simulink model "BD_SER_saber_cosim"  (Simulink 4.1.1)
settings: Solver=ode1  SolverMode=SingleTasking  StartTime=0.0  StopTime=max(cyc_mph(:,1))  FixedStep=1  MaxStep=1  RelTol=1e-3  AbsTol=1e-3
undefined symbols (not defined in the file): cs_fc_off2regen_pwr, cs_fc_spd_setpt_fun, cs_fc_trq_setpt_fun, cs_hi_soc, cs_lo_soc, cyc_mph, ess_max_volts_fun, ess_min_volts_fun, ess_on, ex_calc, fc_emis, fc_map_spd, fc_max_trq, fc_on, fc_spd_scale, fc_trq_scale, fd_ratio, gb_dnshift_load, gb_dnshift_spd, gb_gears_num, gb_num_init, gb_ratio, gb_shift_delay, gb_upshift_load, gb_upshift_spd, gc_map_spd, gc_max_trq, gc_spd_scale, gc_trq_scale, mc_map_spd, mc_max_trq, mc_spd_scale, mc_trq_scale, tc_gc_to_fc_ratio_fun, time_step, tx_speed_dep, vc_idle_bool, vc_idle_spd, wh_radius
libraries: lib_cosimulation x10, lib_outputs x8, lib_controls x5, lib_wheel x2, lib_help x2, lib_transmission x2, lib_accessory x2, lib_interactive x1, lib_drive_cycle x1, lib_exhaust x1, lib_fuel_converter x1, lib_vehicle x1
(part 2 of 2)

== system BD_SER_saber_cosim/Cosimulate Elect/Motor RPM Req/Enabled Subsystem ==
  In1 : Inport  Port=1  LatchInput=off
  Enable : EnablePort
  Out1 : Outport  Port=1
  wires:
  In1/1 -> Out1/1

== system BD_SER_saber_cosim/Cosimulate Elect/Motor Trq Req/Enabled Subsystem ==
  In1 : Inport  Port=1  LatchInput=off
  Enable : EnablePort
  Out1 : Outport  Port=1  InitialOutput=0
  wires:
  In1/1 -> Out1/1

== system BD_SER_saber_cosim/Cosimulate Elect/Series cosim output gotos/Saber_ess2_outputs ==
  In1 : Inport  Port=1  LatchInput=off
  Saber_pb2 : lib_outputs/Saber_pb2
      settings: RTWFcnNameOpts=Auto  RTWFileNameOpts=Auto
  wires:
  In1/1 -> Saber_pb2/1

== system BD_SER_saber_cosim/Cosimulate Elect/Series cosim output gotos/Saber_ess_outputs ==
  In1 : Inport  Port=1  LatchInput=off
  Saber_rint : lib_outputs/Saber_rint
      settings: RTWFcnNameOpts=Auto  RTWFileNameOpts=Auto
  wires:
  In1/1 -> Saber_rint/1

== system BD_SER_saber_cosim/series hybrid control stategy  <cs>/FC on mod/Charge to hi soc: 1 Discharge to lo soc: 0 ==
  In1 : Inport  Port=1  LatchInput=off
  Trigger : TriggerPort  TriggerType=rising  OutputDataType=auto
  Out1 : Outport  Port=1
  wires:
  In1/1 -> Out1/1

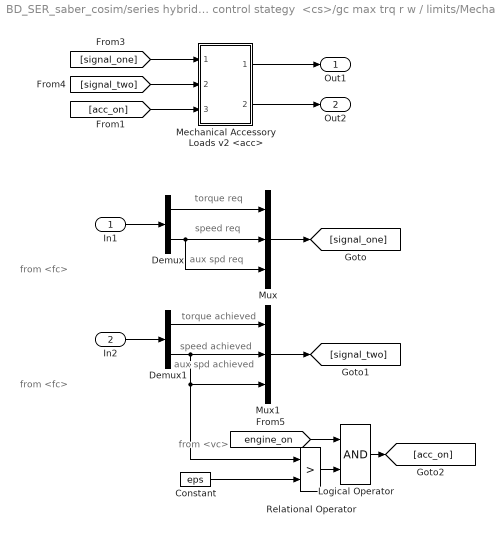
== system BD_SER_saber_cosim/series hybrid control stategy  <cs>/gc max trq r w / limits/Mechanical Accessory Loads <acc> ==
  note: from <fc>
  note: from <fc>
  note: torque req
  note: speed req
  note: aux spd req
  note: torque achieved
  note: speed achieved
  note: aux spd achieved
  note: from <vc>
  In1 : Inport  Port=1  LatchInput=off
  In2 : Inport  Port=2  LatchInput=off
  Constant : Constant  Value=eps
  Demux : Demux  Outputs=2  BusSelectionMode=off
  Demux1 : Demux  Outputs=2  BusSelectionMode=off
  Logical Operator : Logic  Operator=AND  Inputs=2
  Mechanical Accessory Loads v2 <acc> : Subsystem  AncestorBlock=lib_accessory/Mechanical Accessory Loads v2 <acc>  mask{load_on=not(ess_on)*1, acc_max_spd=inf, acc_min_spd=(vc_idle_spd*vc_idle_bool)+eps, ic_mech_trq=0, ic_mech_pwr=0}
      mask prompts: load_on "Electrical Load Status: 1 on; 0 off"; acc_max_spd "maximum shaft speed for aux. (rad/s)"; acc_min_spd "minimum shaft speed for aux. (rad/s)"; ic_mech_trq "Initial Mechanical Torque of the Accessory Loads (Nm)"; ic_mech_pwr "Initial Mechanical Auxiliary Load Power (W)"
      settings: RTWFcnNameOpts=Auto  RTWFileNameOpts=Auto
      mask Display: image(imread('bdi_acc_pic.bmp'))
  Mux : Mux  Inputs=3
  Mux1 : Mux  Inputs=3
  Relational Operator : RelationalOperator  Operator=>
  Out1 : Outport  Port=1
  Out2 : Outport  Port=2
  wires:
  [signal_one] -> Mechanical Accessory Loads v2 <acc>/1("requested shaft T and w, out to the driveline  (Nm ; rad/s; rad/s)")
  Mechanical Accessory Loads v2 <acc>/1("requested shaft and belt T and w, in from the prime mover (Nm ; rad/s)") -> Out1/1
  Mechanical Accessory Loads v2 <acc>/2("achieved shaft T and w, out to the driveline (Nm ; rad/s)") -> Out2/1
  [signal_two] -> Mechanical Accessory Loads v2 <acc>/2("achieved shaft and belt T and w, in from the prime mover (Nm ; rad/s)")
  [acc_on] -> Mechanical Accessory Loads v2 <acc>/3(accessory on/off)
  Mux/1 -> [signal_one]
  In1/1 -> Demux/1
  Demux/1 -> Mux/1
  Demux/2 -> Mux/2, Mux/3
  Mux1/1 -> [signal_two]
  In2/1 -> Demux1/1
  Demux1/1 -> Mux1/1
  Demux1/2 -> Mux1/2, Mux1/3, Relational Operator/1
  Constant/1 -> Relational Operator/2
  [engine_on] -> Logical Operator/1
  Relational Operator/1 -> Logical Operator/2
  Logical Operator/1 -> [acc_on]

== system BD_SER_saber_cosim/<vc> series/gearbox control for series  HV and EV/downshift  command/load fraction ==
  In1 : Inport  Port=1  LatchInput=off
  S-Function : S-Function  FunctionName=sfun_gearbox  Parameters=load, spd  PortCounts=[]  SFunctionModules=''
  Out1 : Outport  Port=1  InitialOutput=0
  wires:
  S-Function/1 -> Out1/1
  In1/1 -> S-Function/1

== system BD_SER_saber_cosim/<vc> series/gearbox control for series  HV and EV/gearbox speed estimator/Block NOTES ==
  note: The requested motor speed is replaced by an estimate of the
      | engine's previous speed whenever the vehicle missed the trace
      |  by more than 1 mph on the last time step.

== system BD_SER_saber_cosim/<vc> series/gearbox control for series  HV and EV/gearbox speed estimator/dt ==
  Clock : Clock
      settings: DisplayTime=off  Decimation=10
  Memory1 : Memory  X0=-1  InheritSampleTime=off
      settings: RTWStateStorageClass=Auto
  Sum4 : Sum  Inputs=+-  SaturateOnIntegerOverflow=on
  Out1 : Outport  Port=1  InitialOutput=0
  wires:
  Clock/1 -> Sum4/1, Memory1/1
  Memory1/1 -> Sum4/2
  Sum4/1 -> Out1/1

== system BD_SER_saber_cosim/<vc> series/gearbox control for series  HV and EV/shifting1/time since last shift ==
  in_1 : Inport  Port=1  LatchInput=off
  just shifted : Subsystem
      settings: RTWFcnNameOpts=Auto  RTWFileNameOpts=Auto
      mask Display: disp('just\nshifted')
  timer : Subsystem
      settings: RTWFcnNameOpts=Auto  RTWFileNameOpts=Auto
      mask Display: disp('timer')
  out_1 : Outport  Port=1  InitialOutput=0
  wires:
  timer/1(time) -> out_1/1
  just shifted/1(out_1) -> timer/1(trigger)
  in_1/1 -> just shifted/1(in_1)

== system BD_SER_saber_cosim/<vc> series/gearbox control for series  HV and EV/upshift  command/load fraction ==
  In1 : Inport  Port=1  LatchInput=off
  S-Function : S-Function  FunctionName=sfun_gearbox  Parameters=load, spd  PortCounts=[]  SFunctionModules=''
  Out1 : Outport  Port=1  InitialOutput=0
  wires:
  S-Function/1 -> Out1/1
  In1/1 -> S-Function/1

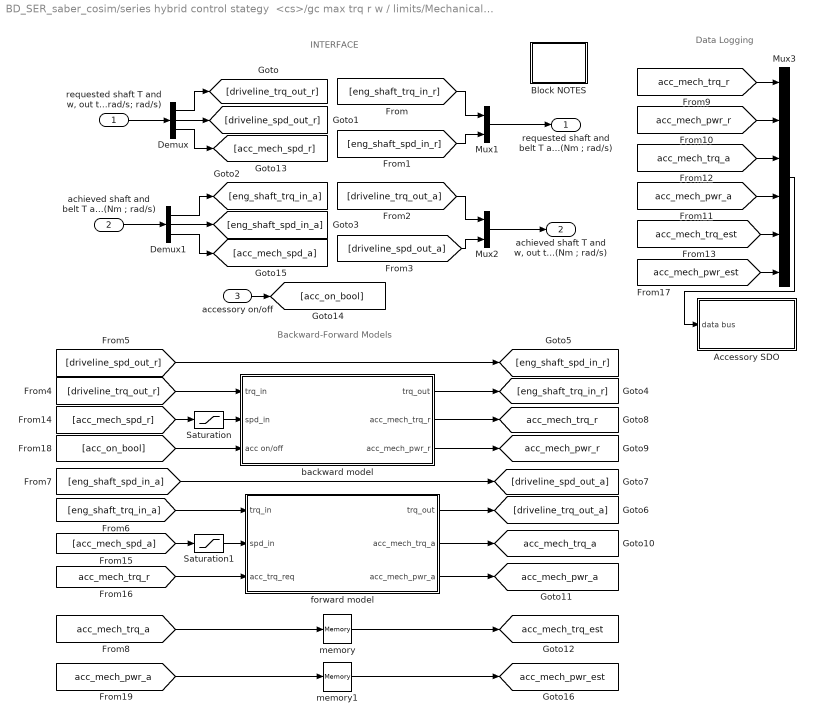
== system BD_SER_saber_cosim/series hybrid control stategy  <cs>/gc max trq r w / limits/Mechanical Accessory Loads <acc>/Mechanical Accessory Loads v2 <acc> ==
  note: Data Logging
  note: Backward-Forward Models
  note: INTERFACE
  "requested shaft T and w, out to the driveline  (Nm ; rad/s; rad/s)" : Inport  Port=1  LatchInput=off
  "achieved shaft and belt T and w, in from the prime mover (Nm ; rad/s)" : Inport  Port=2  LatchInput=off
  accessory on/off : Inport  Port=3  LatchInput=off
  Accessory SDO : Subsystem
      settings: RTWFcnNameOpts=Auto  RTWFileNameOpts=Auto
  Block NOTES : Subsystem
      settings: RTWFcnNameOpts=Auto  RTWFileNameOpts=Auto
      mask Display: disp('Block\nNOTES')
  Demux : Demux  Outputs=3  BusSelectionMode=off
  Demux1 : Demux  Outputs=3  BusSelectionMode=off
  Mux1 : Mux  Inputs=2
  Mux2 : Mux  Inputs=2
  Mux3 : Mux  Inputs=6
  Saturation : Saturate  UpperLimit=acc_max_spd  LowerLimit=acc_min_spd  LinearizeAsGain=on
  Saturation1 : Saturate  UpperLimit=acc_max_spd  LowerLimit=acc_min_spd  LinearizeAsGain=on
  backward model : Subsystem
      settings: RTWFcnNameOpts=Auto  RTWFileNameOpts=Auto
  forward model : Subsystem
      settings: RTWFcnNameOpts=Auto  RTWFileNameOpts=Auto
  memory : Memory  X0=ic_mech_trq  InheritSampleTime=off
      settings: RTWStateStorageClass=Auto
  memory1 : Memory  X0=ic_mech_pwr  InheritSampleTime=off
      settings: RTWStateStorageClass=Auto
  "requested shaft and belt T and w, in from the prime mover (Nm ; rad/s)" : Outport  Port=1
  "achieved shaft T and w, out to the driveline (Nm ; rad/s)" : Outport  Port=2
  tag scope: acc_mech_pwr_a=global, acc_mech_pwr_est=global, acc_mech_pwr_r=global, acc_mech_trq_a=global, acc_mech_trq_est=global, acc_mech_trq_r=global
  wires:
  [acc_mech_pwr_a] -> memory1/1
  [acc_mech_trq_a] -> memory/1
  memory1/1 -> [acc_mech_pwr_est]
  memory/1 -> [acc_mech_trq_est]
  [acc_mech_pwr_est] -> Mux3/6
  Demux/3 -> [acc_mech_spd_r]
  Demux1/3 -> [acc_mech_spd_a]
  [acc_mech_trq_r] -> forward model/3(acc_trq_req)
  Saturation/1 -> backward model/2(spd_in)
  [acc_mech_spd_r] -> Saturation/1
  Saturation1/1 -> forward model/2(spd_in)
  [acc_mech_spd_a] -> Saturation1/1
  forward model/3(acc_mech_pwr_a) -> [acc_mech_pwr_a]
  forward model/2(acc_mech_trq_a) -> [acc_mech_trq_a]
  forward model/1(trq_out) -> [driveline_trq_out_a]
  [acc_on_bool] -> backward model/3(acc on/off)
  accessory on/off/1 -> [acc_on_bool]
  [eng_shaft_trq_in_a] -> forward model/1(trq_in)
  [acc_mech_pwr_a] -> Mux3/4
  [acc_mech_trq_a] -> Mux3/3
  [eng_shaft_spd_in_a] -> [driveline_spd_out_a]
  [driveline_spd_out_r] -> [eng_shaft_spd_in_r]
  [acc_mech_trq_est] -> Mux3/5
  Mux3/1 -> Accessory SDO/1(data bus)
  [acc_mech_pwr_r] -> Mux3/2
  [acc_mech_trq_r] -> Mux3/1
  backward model/1(trq_out) -> [eng_shaft_trq_in_r]
  [driveline_trq_out_r] -> backward model/1(trq_in)
  backward model/3(acc_mech_pwr_r) -> [acc_mech_pwr_r]
  backward model/2(acc_mech_trq_r) -> [acc_mech_trq_r]
  [driveline_spd_out_a] -> Mux2/2
  [driveline_trq_out_a] -> Mux2/1
  Mux2/1 -> "achieved shaft T and w, out to the driveline (Nm ; rad/s)"/1
  [eng_shaft_spd_in_r] -> Mux1/2
  [eng_shaft_trq_in_r] -> Mux1/1
  Mux1/1 -> "requested shaft and belt T and w, in from the prime mover (Nm ; rad/s)"/1
  Demux1/2 -> [eng_shaft_spd_in_a]
  Demux1/1 -> [eng_shaft_trq_in_a]
  "achieved shaft and belt T and w, in from the prime mover (Nm ; rad/s)"/1 -> Demux1/1
  Demux/2 -> [driveline_spd_out_r]
  Demux/1 -> [driveline_trq_out_r]
  "requested shaft T and w, out to the driveline  (Nm ; rad/s; rad/s)"/1 -> Demux/1

== system BD_SER_saber_cosim/<vc> series/gearbox control for series  HV and EV/shifting1/time since last shift/just shifted ==
  in_1 : Inport  Port=1  LatchInput=off
  Memory : Memory  X0=1  InheritSampleTime=off
      settings: RTWStateStorageClass=Auto
  Relational Operator : RelationalOperator  Operator=~=
  out_1 : Outport  Port=1  InitialOutput=0
  wires:
  in_1/1 -> Memory/1, Relational Operator/2
  Memory/1 -> Relational Operator/1
  Relational Operator/1 -> out_1/1

== system BD_SER_saber_cosim/<vc> series/gearbox control for series  HV and EV/shifting1/time since last shift/timer ==
  trigger : Inport  Port=1  LatchInput=off
  Constant : Constant  Value=1
  Constant1 : Constant  Value=0
  Constant2 : Constant  Value=0
  Switch : Switch  Threshold=eps
  no-lag Reset Integrator : Subsystem  mask(No-lag Reset Integrator){@1=15}
      mask prompts: @1 "Initial Value"
      mask help: No-lag Reset Integrator
      mask init:
      | initval=@1;
      settings: RTWFcnNameOpts=Auto  RTWFileNameOpts=Auto
      mask Help: Integrates first input using Euler technique.\nAt the time step that input 2 <> zero,\noutput is reset to input 3.
      mask Display: disp('1/s\nw/ reset\nno lag')
  time : Outport  Port=1  InitialOutput=0
  wires:
  no-lag Reset Integrator/1(out_1) -> Switch/3
  Constant1/1 -> no-lag Reset Integrator/3(in_3)
  Constant/1 -> no-lag Reset Integrator/1(in_1)
  Constant2/1 -> Switch/1
  trigger/1 -> no-lag Reset Integrator/2(in_2), Switch/2
  Switch/1 -> time/1

== system BD_SER_saber_cosim/series hybrid control stategy  <cs>/gc max trq r w / limits/Mechanical Accessory Loads <acc>/Mechanical Accessory Loads v2 <acc>/Accessory SDO ==
  data bus : Inport  Port=1  LatchInput=off
  Demux : Demux  Outputs=6  BusSelectionMode=off
  To Workspace : ToWorkspace  VariableName=acc_mech_trq_r  SampleTime=-1  SaveFormat=Array
  To Workspace1 : ToWorkspace  VariableName=acc_mech_pwr_a  SampleTime=-1  SaveFormat=Array
  To Workspace2 : ToWorkspace  VariableName=acc_mech_trq_est  SampleTime=-1  SaveFormat=Array
  To Workspace3 : ToWorkspace  VariableName=acc_mech_pwr_r  SampleTime=-1  SaveFormat=Array
  To Workspace4 : ToWorkspace  VariableName=acc_mech_trq_a  SampleTime=-1  SaveFormat=Array
  To Workspace5 : ToWorkspace  VariableName=acc_mech_pwr_est  SampleTime=-1  SaveFormat=Array
  mechanical power logging : lib_accessory/SubLibraries/mechanical power logging  eff=acc_mech_eff
  wires:
  Demux/6 -> To Workspace5/1
  Demux/5 -> To Workspace2/1
  Demux/3 -> To Workspace4/1
  Demux/2 -> To Workspace3/1
  Demux/1 -> To Workspace/1
  Demux/4 -> To Workspace1/1, mechanical power logging/1
  data bus/1 -> Demux/1

== system BD_SER_saber_cosim/series hybrid control stategy  <cs>/gc max trq r w / limits/Mechanical Accessory Loads <acc>/Mechanical Accessory Loads v2 <acc>/Block NOTES ==
  note: In this model, only one speed is used to predict accessory
      | loading. The forward model is "dummied" out.
  note: A third input is given for accessory load speed. This is done so that
      | the accessory block can use fc_spd_est which is an estimated vehicle speed
      | (equal to fc_spd_out under normal circumstances).
      | Using fc_spd_est provides total compatibility with ADVISOR v3.2
  note: In terms of an interface, the model assumes belt-driven mechanical loads
      | that run off of a prime mover shaft (e.g., engine shaft)
      |
      | This model takes in requested driveline torque and speed requests and
      | augments torque due to belt driven accessories.
      |
      | The torque passed along down to the driveline is only torque to move the
      | vehicle.
  note: This is the mechanical auxiliary loads model.

== system BD_SER_saber_cosim/series hybrid control stategy  <cs>/gc max trq r w / limits/Mechanical Accessory Loads <acc>/Mechanical Accessory Loads v2 <acc>/backward model ==
  note: Power, W, input to accessory
  note: T, Nm, shaft out
  note: T, Nm, driveline
  note: T, Nm, accessory
  note: w_apu, rad/s
  trq_in : Inport  Port=1  LatchInput=off
  spd_in : Inport  Port=2  LatchInput=off
  acc on/off : Inport  Port=3  LatchInput=off
  Product : Product  Inputs=**  Multiplication=Element-wise(.*)  SaturateOnIntegerOverflow=on
  Product1 : Product  Inputs=**  Multiplication=Element-wise(.*)  SaturateOnIntegerOverflow=on
  Sum : Sum  Inputs=|++  SaturateOnIntegerOverflow=on
  acc_mech_var_loads : ToWorkspace  VariableName=acc_mech_var_load  SampleTime=-1  SaveFormat=Structure
  mechanical accessories (Nm) : Subsystem  BlockChoice=Mechanical Accessories: Speed Dependant and Variable Electrical
      settings: AttributesFormatString=%<BlockChoice>  TemplateBlock=lib_accessory/mechanical accessories (Nm)  MemberBlocks=Mechanical Accessories: Const Mech Var Elect,Mechanical Accessories: Constant Mechanical & Electrical,Mechanical Accessories: Speed Dependant and Variable Electrical,Saber Dual Voltage Cosim,Saber Single Voltage Cosim,SindaTransAC  RTWFcnNameOpts=Auto  RTWFileNameOpts=Auto
      mask Display: image(imread('bdi_acc_pic_cs.bmp'))
  trq_out : Outport  Port=1
  acc_mech_trq_r : Outport  Port=2
  acc_mech_pwr_r : Outport  Port=3
  wires:
  mechanical accessories (Nm)/3(probes) -> acc_mech_var_loads/1
  [acc_on] -> Product1/2
  [acc_on] -> Product/1
  acc on/off/1 -> [acc_on]
  mechanical accessories (Nm)/2(P_mech_acc) -> Product1/1
  Product1/1 -> acc_mech_pwr_r/1
  mechanical accessories (Nm)/1(T_acc) -> Product/2
  Product/1 -> Sum/2, acc_mech_trq_r/1
  Sum/1 -> trq_out/1
  trq_in/1 -> Sum/1
  spd_in/1 -> mechanical accessories (Nm)/1(w_APU)

== system BD_SER_saber_cosim/series hybrid control stategy  <cs>/gc max trq r w / limits/Mechanical Accessory Loads <acc>/Mechanical Accessory Loads v2 <acc>/forward model ==
  note: acc torque, Nm
  note: NOTES
  note: This simplistic model may not correctly account for accessory torque and/or power
      | when the upstream torque provider is torque or speed limited
  note: Power, W, input to accessory
  note: T, Nm, shaft out
  note: driveline and
      | acc torque, Nm
  note: T, Nm, accessory
  note: acc speed, rad/s
  trq_in : Inport  Port=1  LatchInput=off
  spd_in : Inport  Port=2  LatchInput=off
  acc_trq_req : Inport  Port=3  LatchInput=off
  Product1 : Product  Inputs=**  Multiplication=Element-wise(.*)  SaturateOnIntegerOverflow=on
  Sum : Sum  Inputs=|+-  SaturateOnIntegerOverflow=on
  trq_out : Outport  Port=1
  acc_mech_trq_a : Outport  Port=2
  acc_mech_pwr_a : Outport  Port=3
  wires:
  [pm_trq_a] -> Sum/1
  acc_trq_req/1 -> [acc_trq_r]
  trq_in/1 -> [pm_trq_a]
  [acc_spd] -> Product1/2
  [acc_trq_r] -> Product1/1, Sum/2, acc_mech_trq_a/1
  Product1/1 -> acc_mech_pwr_a/1
  Sum/1 -> trq_out/1
  spd_in/1 -> [acc_spd]

== system BD_SER_saber_cosim/<vc> series/gearbox control for series  HV and EV/shifting1/time since last shift/timer/no-lag Reset Integrator ==
  in_1 : Inport  Port=1  LatchInput=off
  in_2 : Inport  Port=2  LatchInput=off
  in_3 : Inport  Port=3  LatchInput=off
  Constant : Constant  Orientation=up  Value=0
  Memory : Memory  Orientation=left  X0=initval  InheritSampleTime=off
      settings: RTWStateStorageClass=Auto
  Product : Product  Inputs=2  Multiplication=Element-wise(.*)  SaturateOnIntegerOverflow=on
  Sum : Sum  Inputs=++  SaturateOnIntegerOverflow=on
  Switch : Switch  Threshold=eps
  dt : Subsystem  Orientation=down
      settings: RTWFcnNameOpts=Auto  RTWFileNameOpts=Auto
  in_2==0 : RelationalOperator  Operator===
  out_1 : Outport  Port=1  InitialOutput=0
  wires:
  Constant/1 -> in_2==0/2
  in_2==0/1 -> Switch/2
  Switch/1 -> Memory/1, out_1/1
  Sum/1 -> Switch/1
  Memory/1 -> Sum/1
  Product/1 -> Sum/2
  dt/1(out_1) -> Product/1
  in_1/1 -> Product/2
  in_2/1 -> in_2==0/1
  in_3/1 -> Switch/3

== system BD_SER_saber_cosim/series hybrid control stategy  <cs>/gc max trq r w / limits/Mechanical Accessory Loads <acc>/Mechanical Accessory Loads v2 <acc>/backward model/mechanical accessories (Nm) ==
  w_APU : Inport  Port=1  LatchInput=off
  Mechanical Accessories: Speed Dependant and Variable Electrical : lib_accessory/Mechanical Accessories: Speed Dependant and Variable Electrical
  T_acc : Outport  Port=1
  P_mech_acc : Outport  Port=2
  probes : Outport  Port=3
  wires:
  w_APU/1 -> Mechanical Accessories: Speed Dependant and Variable Electrical/1
  Mechanical Accessories: Speed Dependant and Variable Electrical/1 -> T_acc/1
  Mechanical Accessories: Speed Dependant and Variable Electrical/2 -> P_mech_acc/1
  Mechanical Accessories: Speed Dependant and Variable Electrical/3 -> probes/1

== system BD_SER_saber_cosim/<vc> series/gearbox control for series  HV and EV/shifting1/time since last shift/timer/no-lag Reset Integrator/dt ==
  Clock : Clock
      settings: DisplayTime=off  Decimation=10
  Memory1 : Memory  X0=-1  InheritSampleTime=off
      settings: RTWStateStorageClass=Auto
  Sum1 : Sum  Inputs=+-  SaturateOnIntegerOverflow=on
  out_1 : Outport  Port=1  InitialOutput=0
  wires:
  Sum1/1 -> out_1/1
  Memory1/1 -> Sum1/2
  Clock/1 -> Memory1/1, Sum1/1
